simulink model "CruiseControl_Req"  (R2020a)
settings: configuration reference "ModelReferencingVisual" (kept outside this file)
values from neighbouring files (symbols this model uses):
  holdrate = 5.0    [CruiseControl_Req_dd.sldd]
  incdec = 1.0    [CruiseControl_Req_dd.sldd]
  maxtspeed = 90.0    [CruiseControl_Req_dd.sldd]
  mintspeed = 20.0    [CruiseControl_Req_dd.sldd]
settings Model: DataDictionary=CruiseControl_Req_dd.sldd  EnableAccessToBaseWorkspace=off  Creator=The MathWorks Inc.  LastModifiedBy=promero
settings ConfigSetRef: SourceName=ModelReferencingVisual

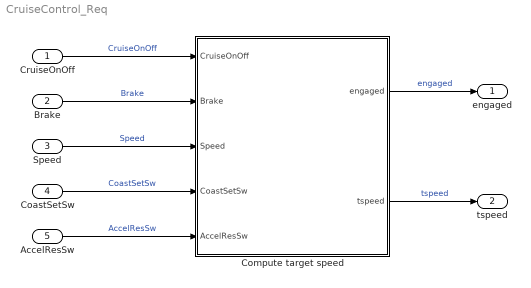
== system CruiseControl_Req ==
  CruiseOnOff : Inport  PortDimensions=1
  Brake : Inport  Port=2  PortDimensions=1
  Speed : Inport  Port=3  PortDimensions=1
  CoastSetSw : Inport  Port=4  PortDimensions=1
  AccelResSw : Inport  Port=5  PortDimensions=1
  Compute target speed : Stateflow chart  TreatAsAtomicUnit=on
  engaged : Outport  VectorParamsAs1DForOutWhenUnconnected=off
  tspeed : Outport  Port=2  VectorParamsAs1DForOutWhenUnconnected=off
  wires:
  AccelResSw/1 -> Compute target speed/5(AccelResSw)  "AccelResSw"
  Speed/1 -> Compute target speed/3(Speed)  "Speed"
  CoastSetSw/1 -> Compute target speed/4(CoastSetSw)  "CoastSetSw"
  CruiseOnOff/1 -> Compute target speed/1(CruiseOnOff)  "CruiseOnOff"
  Brake/1 -> Compute target speed/2(Brake)  "Brake"
  Compute target speed/1(engaged) -> engaged/1  "engaged"
  Compute target speed/2(tspeed) -> tspeed/1  "tspeed"

== stateflow chart CruiseControl_Req/Compute target speed ==
  state OFF
    en:
    engaged = false;
    tspeed = 0;
  state CRUISE
    state ON
      en: engaged = true;
      state Accel
        entry: tspeed = tspeed - incdec;
      state Steady
      state Coast
        entry: tspeed = tspeed - incdec;
      (junction 60) -> Accel
      (junction 57) -> (junction 60) : [after(10/holdrate...
          | *incdec,tick)]
      Accel -> (junction 57) [order 1]
      Steady -> Accel [order 1] : [hasChangedTo(AccelResSw,true) ...
          | && tspeed < maxtspeed]
      Accel -> Steady [order 2] : [!AccelResSw || ...
          | tspeed > maxtspeed]
      Steady -> (junction 75) [order 3] : [hasChangedTo(CoastSetSw,true)]
      (default) -> (junction 75)
      (junction 75) -> (junction 77) : {tspeed = Speed;}
      (junction 77) -> Steady
      Steady -> Coast [order 2] : [hasChangedTo(CoastSetSw,true) ...
          | && tspeed > mintspeed]
      Coast -> Steady [order 2] : [!CoastSetSw || ...
          | tspeed < mintspeed]
      (junction 72) -> Coast
      (junction 71) -> (junction 72) : [after(10/holdrate...
          | *incdec,tick)]
      Coast -> (junction 71) [order 1]
    state STANDBY
      en:
      engaged=false;
    (default) -> STANDBY
    ON -> STANDBY : [Brake||Speed> maxtspeed||Speed<mintspeed]
    STANDBY -> (junction 103) : [~Brake && ...
        | Speed<=maxtspeed && ...
        | Speed>=mintspeed]
    (junction 103) -> Steady [order 1] : [hasChangedTo(AccelResSw,true)...
        | &&tspeed!=0]
    (junction 103) -> (junction 106) [order 2]
    (junction 106) -> ON : [hasChangedTo(CoastSetSw,true)]
  (default) -> OFF
  OFF -> CRUISE : [CruiseOnOff]
  CRUISE -> OFF : [~CruiseOnOff]
  data: engaged output boolean; CruiseOnOff input; Brake input; Speed input; CoastSetSw input; AccelResSw input; tspeed output uint8; incdec parameter; holdrate parameter; maxtspeed parameter; mintspeed parameter
